simulink model "aocs_plant"  (R2025a)
settings: Solver=ode45  StartTime=0  StopTime=200  RelTol=1e-09  AbsTol=1e-10
undefined symbols (not defined in the file): AOCS, AOCS_Config, AOCS_EnvironmentConfig, AOCS_GNCConfig, AOCS_OrbitConfig, AOCS_SensorConfig, IAU, juliandate, propagateOnboardSgp4
libraries: aerolibtransform2 x8, simulink x8, matrix_library x5
(part 3 of 3)

== system aocs_plant/Flight Dynamics/Orbit & Environment/Environment Products/Atmosphere Products/Atmosphere Model ==
  EnvironmentConfig : Inport  OutDataTypeStr=Bus: EnvironmentConfigBus
  OrbitState : Inport  Port=2  OutDataTypeStr=Bus: OrbitStateBus
  lla : Inport  Port=3  OutDataTypeStr=double
  EnvironmentContext : Inport  Port=4  OutDataTypeStr=Bus: EnvironmentContextBus
  Atmosphere Bus Assembly : BusCreator  Inputs=12  OutDataTypeStr=Bus: AtmosphereBus  NonVirtualBus=on
  Atmosphere Products : Subsystem
  Select Orbit State : BusSelector  OutputSignals=r_I_m,v_I_m_s
  Atmosphere : Outport  OutDataTypeStr=Bus: AtmosphereBus
  wires:
  OrbitState/1 -> Select Orbit State/1
  Atmosphere Bus Assembly/1 -> Atmosphere/1
  Select Orbit State/1 -> Atmosphere Products/1(r_I_m)  "<r_I_m>"
  Select Orbit State/2 -> Atmosphere Products/2(v_I_m_s)  "<v_I_m_s>"
  lla/1 -> Atmosphere Products/3(lla)
  EnvironmentConfig/1 -> Atmosphere Products/4(EnvironmentConfig)
  EnvironmentContext/1 -> Atmosphere Products/5(EnvironmentContext)
  Atmosphere Products/1(rho_kg_m3) -> Atmosphere Bus Assembly/1
  Atmosphere Products/2(rho_raw_kg_m3) -> Atmosphere Bus Assembly/2
  Atmosphere Products/3(rho_uncertainty_1sigma_kg_m3) -> Atmosphere Bus Assembly/3
  Atmosphere Products/4(T_local_K) -> Atmosphere Bus Assembly/4
  Atmosphere Products/5(T_exo_K) -> Atmosphere Bus Assembly/5
  Atmosphere Products/6(n_O_m3) -> Atmosphere Bus Assembly/6
  Atmosphere Products/7(n_N2_m3) -> Atmosphere Bus Assembly/7
  Atmosphere Products/8(n_O2_m3) -> Atmosphere Bus Assembly/8
  Atmosphere Products/9(n_He_m3) -> Atmosphere Bus Assembly/9
  Atmosphere Products/10(n_H_m3) -> Atmosphere Bus Assembly/10
  Atmosphere Products/11(n_N_m3) -> Atmosphere Bus Assembly/11
  Atmosphere Products/12(v_atm_I_m_s) -> Atmosphere Bus Assembly/12

== system aocs_plant/Flight Dynamics/Orbit & Environment/Environment Products/Atmosphere Products/Frame Transformations ==
  In1 : Inport
  In2 : Inport  Port=2
  Clock : Clock
  Clock2 : Clock
  Direction Cosine Matrix ECI to ECEF1 : aerolibtransform2/Direction Cosine Matrix ECI to ECEF  red=IAU-2000/2006  year=2026  month=January  day=1  hour=0  min=0  sec=0  deltaT=Sec  errorflag=Error  extraparamflag=on
      settings: AttributesFormatString=%<red>
  ECI Position to LLA : aerolibtransform2/ECI Position to LLA  red=IAU-2000/2006  year=2026  month=January  day=1  hour=0  min=0  sec=0  deltaT=Sec  errorflag=Error  extraparamflag=on  eunits=Metric (MKS)  earthmodel=WGS84  flat=1/298.257223563  eqradius=6378137
      settings: AttributesFormatString=%<red>
  MATLAB Function : MATLAB Function  TreatAsAtomicUnit=on
  Select Environment Context : BusSelector  OutputSignals=delta_ut1_s,delta_at_s,polar_motion_rad,d_cip_rad
  Select Orbit State : BusSelector  OutputSignals=v_I_m_s,r_I_m
  Terminator : Terminator
  lla : Outport
  v_ECEF_m_s : Outport  Port=2
  C_ECEF_ECI : Outport  Port=3
  wires:
  In2/1 -> Select Environment Context/1
  ECI Position to LLA/1 -> lla/1
  Clock2/1 -> Direction Cosine Matrix ECI to ECEF1/5  "sec"
  Select Environment Context/2 -> Direction Cosine Matrix ECI to ECEF1/2, ECI Position to LLA/3  "<delta_at_s>"
  Select Orbit State/2 -> MATLAB Function/2(r_I_m), ECI Position to LLA/1  "<r_I_m>"
  In1/1 -> Select Orbit State/1
  Select Environment Context/4 -> Direction Cosine Matrix ECI to ECEF1/4, ECI Position to LLA/5  "<d_cip_rad>"
  Select Environment Context/1 -> Direction Cosine Matrix ECI to ECEF1/1, ECI Position to LLA/2  "<delta_ut1_s>"
  Clock/1 -> ECI Position to LLA/6  "sec"
  Select Environment Context/3 -> ECI Position to LLA/4, Direction Cosine Matrix ECI to ECEF1/3  "<polar_motion_rad>"
  Direction Cosine Matrix ECI to ECEF1/1 -> MATLAB Function/3(C_ECEF_ECI), C_ECEF_ECI/1  "C_ECEF_ECI"
  Select Orbit State/1 -> MATLAB Function/1(v_I_m_s)  "<v_I_m_s>"
  MATLAB Function/2(v_ECEF_m_s) -> v_ECEF_m_s/1
  MATLAB Function/1(r_E_m) -> Terminator/1

== system aocs_plant/Flight Dynamics/Orbit & Environment/Orbit Propagator & Time/Orbit State/Orbit Propagator ==
  OrbitAcceleration : Inport
  Bus Creator : BusCreator  Inputs=2
  Orbit Propagator Kepler (unperturbed) : OrbitPropagator  propagator=Numerical (high precision)  accelIn=on  startDate=AOCS_OrbitConfig.epoch_utc  action=None  semiMajorAxis=AOCS_OrbitConfig.semi_major_axis_m  eccentricity=AOCS_OrbitConfig.eccentricity  inclination=AOCS_OrbitConfig.inclination_rad  raan=AOCS_OrbitConfig.raan_rad  argPeriapsis=AOCS_OrbitConfig.argument_of_periapsis_rad  trueAnomaly=AOCS_OrbitConfig.true_anomaly_rad  inertialPosition=[3649700.0 3308200.0 -4676600.0]  inertialVelocity=[-2750.8 6666.4 2573.4]  fixedPosition=[-4142689.0 -2676864.7 -4669861.6]  fixedVelocity=[1452.7 -6720.7 2568.1]  customR=3396200  customMu=4.305e13  customJ2=1.0826269e-03  customOmega=4.06125949e-3  ephemerisStartDate=[2020 1 1 0 0 0]  ephemerisEndDate=[2030 1 1 0 0 0]  useThirdBodyGravity=on  angleUnits=Radians  timeFormat=Gregorian date
  Terminator : Terminator
  OrbitState : Outport  OutDataTypeStr=Bus: OrbitStateBus
  wires:
  Orbit Propagator Kepler (unperturbed)/3 -> Terminator/1
  Bus Creator/1 -> OrbitState/1
  Orbit Propagator Kepler (unperturbed)/1 -> Bus Creator/1  "r_I_m"
  Orbit Propagator Kepler (unperturbed)/2 -> Bus Creator/2  "v_I_m_s"
  OrbitAcceleration/1 -> Orbit Propagator Kepler (unperturbed)/1

== system aocs_plant/Sensors/GNSS/PVT Error Model/Position Error RTN/Gauss-Markov ==
  Innovation Std : Gain  Gain=diag(AOCS_SensorConfig.GNSS.position_gauss_markov_step_std_RTN_m)  Multiplication=Matrix(K*u)
  Innovation W : RandomNumber  Mean=zeros(3,1)  Variance=ones(3,1)  Seed=AOCS_SensorConfig.GNSS.position_gauss_markov_seed  SampleTime=AOCS_SensorConfig.GNSS.sample_time_s
  State Delay : UnitDelay  InitialCondition=zeros(3,1)  SampleTime=AOCS_SensorConfig.GNSS.sample_time_s  HasFrameUpgradeWarning=on
  State Transition : Gain  Gain=AOCS_SensorConfig.GNSS.gauss_markov_alpha
  State Update : Sum
  state : Outport
  wires:
  Innovation W/1 -> Innovation Std/1
  Innovation Std/1 -> State Update/1
  State Delay/1 -> State Transition/1
  State Transition/1 -> State Update/2
  State Update/1 -> State Delay/1, state/1  "state"

== system aocs_plant/Sensors/GNSS/PVT Error Model/Velocity Error RTN/Gauss-Markov ==
  Innovation Std : Gain  Gain=diag(AOCS_SensorConfig.GNSS.velocity_gauss_markov_step_std_RTN_m_s)  Multiplication=Matrix(K*u)
  Innovation W : RandomNumber  Mean=zeros(3,1)  Variance=ones(3,1)  Seed=AOCS_SensorConfig.GNSS.velocity_gauss_markov_seed  SampleTime=AOCS_SensorConfig.GNSS.sample_time_s
  State Delay : UnitDelay  InitialCondition=zeros(3,1)  SampleTime=AOCS_SensorConfig.GNSS.sample_time_s  HasFrameUpgradeWarning=on
  State Transition : Gain  Gain=AOCS_SensorConfig.GNSS.gauss_markov_alpha
  State Update : Sum
  state : Outport
  wires:
  Innovation W/1 -> Innovation Std/1
  Innovation Std/1 -> State Update/1
  State Delay/1 -> State Transition/1
  State Transition/1 -> State Update/2
  State Update/1 -> State Delay/1, state/1  "state"

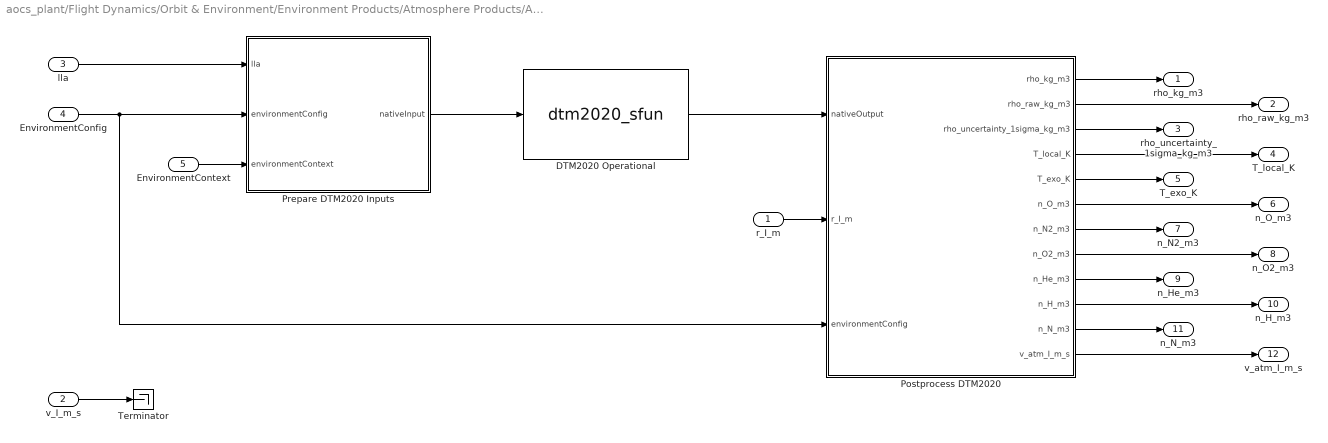
== system aocs_plant/Flight Dynamics/Orbit & Environment/Environment Products/Atmosphere Products/Atmosphere Model/Atmosphere Products ==
  r_I_m : Inport
  v_I_m_s : Inport  Port=2
  lla : Inport  Port=3
  EnvironmentConfig : Inport  Port=4
  EnvironmentContext : Inport  Port=5
  DTM2020 Operational : S-Function  FunctionName=dtm2020_sfun  Parameters=AOCS_DTM2020_CoefficientFile  SFunctionDeploymentMode=off  EnableBusSupport=off
  Postprocess DTM2020 : MATLAB Function  TreatAsAtomicUnit=on
  Prepare DTM2020 Inputs : MATLAB Function  TreatAsAtomicUnit=on
  Terminator : Terminator
  rho_kg_m3 : Outport
  rho_raw_kg_m3 : Outport  Port=2
  rho_uncertainty_1sigma_kg_m3 : Outport  Port=3
  T_local_K : Outport  Port=4
  T_exo_K : Outport  Port=5
  n_O_m3 : Outport  Port=6
  n_N2_m3 : Outport  Port=7
  n_O2_m3 : Outport  Port=8
  n_He_m3 : Outport  Port=9
  n_H_m3 : Outport  Port=10
  n_N_m3 : Outport  Port=11
  v_atm_I_m_s : Outport  Port=12
  wires:
  lla/1 -> Prepare DTM2020 Inputs/1(lla)
  EnvironmentConfig/1 -> Postprocess DTM2020/3(environmentConfig), Prepare DTM2020 Inputs/2(environmentConfig)
  EnvironmentContext/1 -> Prepare DTM2020 Inputs/3(environmentContext)
  Prepare DTM2020 Inputs/1(nativeInput) -> DTM2020 Operational/1
  DTM2020 Operational/1 -> Postprocess DTM2020/1(nativeOutput)
  r_I_m/1 -> Postprocess DTM2020/2(r_I_m)
  Postprocess DTM2020/1(rho_kg_m3) -> rho_kg_m3/1
  Postprocess DTM2020/2(rho_raw_kg_m3) -> rho_raw_kg_m3/1
  Postprocess DTM2020/3(rho_uncertainty_1sigma_kg_m3) -> rho_uncertainty_1sigma_kg_m3/1
  Postprocess DTM2020/4(T_local_K) -> T_local_K/1
  Postprocess DTM2020/5(T_exo_K) -> T_exo_K/1
  Postprocess DTM2020/6(n_O_m3) -> n_O_m3/1
  Postprocess DTM2020/7(n_N2_m3) -> n_N2_m3/1
  Postprocess DTM2020/8(n_O2_m3) -> n_O2_m3/1
  Postprocess DTM2020/9(n_He_m3) -> n_He_m3/1
  Postprocess DTM2020/10(n_H_m3) -> n_H_m3/1
  Postprocess DTM2020/11(n_N_m3) -> n_N_m3/1
  Postprocess DTM2020/12(v_atm_I_m_s) -> v_atm_I_m_s/1
  v_I_m_s/1 -> Terminator/1

== matlab function aocs_plant/Flight Dynamics/Orbit & Environment/Environment Products/Atmosphere Products/Atmosphere Model/Atmosphere Products/Postprocess DTM2020 ==
  data: nativeOutput input; rho_kg_m3 output; r_I_m input; environmentConfig input; rho_raw_kg_m3 output; rho_uncertainty_1sigma_kg_m3 output; T_local_K output; T_exo_K output; n_O_m3 output; n_N2_m3 output; n_O2_m3 output; n_He_m3 output; n_H_m3 output; n_N_m3 output; v_atm_I_m_s output
function [rho_kg_m3, rho_raw_kg_m3, rho_uncertainty_1sigma_kg_m3, ...
    T_local_K, T_exo_K, n_O_m3, n_N2_m3, n_O2_m3, n_He_m3, ...
    n_H_m3, n_N_m3, v_atm_I_m_s] = postprocessDtm(nativeOutput, r_I_m, environmentConfig)
%#codegen
[rho_kg_m3, rho_raw_kg_m3, rho_uncertainty_1sigma_kg_m3, ...
    T_local_K, T_exo_K, n_O_m3, n_N2_m3, n_O2_m3, n_He_m3, ...
    n_H_m3, n_N_m3, v_atm_I_m_s] = dtm2020.postprocessNativeOutput( ...
    nativeOutput, r_I_m, environmentConfig);
end

== matlab function aocs_plant/Sensors/Coarse Sun Sensors/Coarse Sun Sensor Model ==
  data: sun_B_unit input; sun_B_unit_meas output; solar_flux_shadowed_W_m2 input; sun_visibility input; css input; noise_unit input; irradiance_W_m2 output; panel_signals_W_m2 output; valid output
function [sun_B_unit_meas, irradiance_W_m2, panel_signals_W_m2, valid] = coarseSunSensors(sun_B_unit, solar_flux_shadowed_W_m2, sun_visibility, css, noise_unit)
%#codegen
panel_cosines = css.panel_normals_B.' * normalizeVector(sun_B_unit, [1.0; 0.0; 0.0]);
visible = panel_cosines >= css.fov_cos;
ideal_panel_signals_W_m2 = solar_flux_shadowed_W_m2 .* max(panel_cosines, 0.0) .* double(visible);
panel_signals_W_m2 = (1.0 + css.scale_factor) .* ideal_panel_signals_W_m2 + css.bias_W_m2 + css.noise_std_W_m2 .* noise_unit;
panel_signals_W_m2 = min(max(panel_signals_W_m2, 0.0), css.range_W_m2);
if css.resolution_W_m2 > 0.0
    panel_signals_W_m2 = round(panel_signals_W_m2 ./ css.resolution_W_m2) .* css.resolution_W_m2;
end

sun_raw_B = [
    panel_signals_W_m2(1) - panel_signals_W_m2(2);
    panel_signals_W_m2(3) - panel_signals_W_m2(4);
    panel_signals_W_m2(5) - panel_signals_W_m2(6)];
sun_B_unit_meas = normalizeVector(sun_raw_B, [1.0; 0.0; 0.0]);
irradiance_W_m2 = max(panel_signals_W_m2);
valid = double(css.enabled > 0.5 && sun_visibility > 0.5 && irradiance_W_m2 >= css.min_valid_irradiance_W_m2);

if css.mode_id == 2.0
    panel_signals_W_m2 = css.failure_panel_signals_W_m2;
    sun_B_unit_meas = normalizeVector(css.failure_sun_B_unit, [1.0; 0.0; 0.0]);
    irradiance_W_m2 = css.failure_irradiance_W_m2;
    valid = double(css.failure_valid > 0.5);
end

if css.enabled <= 0.5
    panel_signals_W_m2 = zeros(6, 1);
    sun_B_unit_meas = [1.0; 0.0; 0.0];
    irradiance_W_m2 = 0.0;
    valid = 0.0;
end
end

function unitVector = normalizeVector(vector, defaultVector)
normVector = norm(vector);
if normVector <= 1.0e-12
    unitVector = defaultVector;
else
    unitVector = vector ./ normVector;
end
end

== matlab function aocs_plant/Sensors/GNSS/PVT Error Model/Apply RTN Errors ==
  data: rTruth_I_m input; rMeasured_I_m output; vTruth_I_m_s input; positionError_RTN_m input; velocityError_RTN_m_s input; vMeasured_I_m_s output
function [rMeasured_I_m, vMeasured_I_m_s] = applyRtnErrors(rTruth_I_m, vTruth_I_m_s, positionError_RTN_m, velocityError_RTN_m_s)
%#codegen
[rMeasured_I_m, vMeasured_I_m_s] = applyGnssRtnErrors(rTruth_I_m, vTruth_I_m_s, positionError_RTN_m, velocityError_RTN_m_s);
end

== matlab function aocs_plant/Flight Dynamics/Orbit & Environment/Disturbance Torques/Gravity Gradient Path/Gravity Gradient Torque ==
  data: r_I_m input; M_gg_B_Nm output; DCM_be input; I_B input; mu_m3_s2 input
function M_gg_B_Nm = gravityGradientTorque(r_I_m, DCM_be, I_B, mu_m3_s2)
r_norm_m = norm(r_I_m);

if r_norm_m <= 0
    M_gg_B_Nm = zeros(3,1);
    return;
end

r_hat_I = r_I_m / r_norm_m;
r_hat_B = DCM_be * r_hat_I;

M_gg_B_Nm = 3 * mu_m3_s2 / r_norm_m^3 * cross(r_hat_B, I_B * r_hat_B);
end

== matlab function aocs_plant/Flight Dynamics/Orbit & Environment/Disturbance Torques/Aerodynamic Disturbance Path/Relative Wind/Relative Wind Products ==
  data: v_I_m_s input; v_flow_B_m_s output; v_atm_I_m_s input; DCM_be input; rho_kg_m3 input; v_rel_norm_m_s output; q_dyn_N_m2 output
function [v_flow_B_m_s, v_rel_norm_m_s, q_dyn_N_m2] = ...
    relativeWindProducts(v_I_m_s, v_atm_I_m_s, DCM_be, rho_kg_m3)
%#codegen

v_rel_I_m_s = v_I_m_s(:) - v_atm_I_m_s(:);
v_flow_B_m_s = -DCM_be * v_rel_I_m_s;
v_rel_norm_m_s = norm(v_rel_I_m_s);
q_dyn_N_m2 = 0.5 * max(rho_kg_m3, 0.0) * v_rel_norm_m_s^2;
end

== matlab function aocs_plant/Flight Dynamics/Orbit & Environment/Disturbance Torques/Aerodynamic Disturbance Path/Sentman Multispecies Panels ==
  data: v_flow_B_m_s input; F_aero_B_N output; rho_kg_m3 input; T_local_K input; number_densities_m3 input; C_BI input; mass_kg input; aero_enabled input; panel_normals_B input; panel_areas_m2 input; panel_centers_B_m input; wall_temperature_K input; energy_accommodation input; M_aero_B_Nm output; F_aero_I_N output; a_aero_I_m_s2 output; panel_forces_B_N output; q_dyn_N_m2 output
function [F_aero_B_N, M_aero_B_Nm, F_aero_I_N, a_aero_I_m_s2, ...
    panel_forces_B_N, q_dyn_N_m2] = sentmanPanels(v_flow_B_m_s, rho_kg_m3, ...
    T_local_K, number_densities_m3, C_BI, mass_kg, aero_enabled, ...
    panel_normals_B, panel_areas_m2, panel_centers_B_m, ...
    wall_temperature_K, energy_accommodation)
%#codegen
[F_aero_B_N, M_aero_B_Nm, F_aero_I_N, a_aero_I_m_s2, ...
    panel_forces_B_N, q_dyn_N_m2] = computeSentmanPanelAerodynamics( ...
    v_flow_B_m_s, rho_kg_m3, T_local_K, number_densities_m3, C_BI, ...
    mass_kg, aero_enabled, panel_normals_B, panel_areas_m2, ...
    panel_centers_B_m, wall_temperature_K, energy_accommodation);
end

== matlab function aocs_plant/Flight Dynamics/Orbit & Environment/Disturbance Torques/SRP Disturbance Path/SRP Inertial Acceleration ==
  data: F_srp_B_N input; F_srp_I_N output; C_BI input; mass_kg input; a_srp_I_m_s2 output
function [F_srp_I_N, a_srp_I_m_s2] = srpAcceleration(F_srp_B_N, C_BI, mass_kg)
%#codegen
[F_srp_I_N, a_srp_I_m_s2] = computeSrpAcceleration(F_srp_B_N, C_BI, mass_kg);
end

== matlab function aocs_plant/Flight Dynamics/Numerical Checks/Finite Values ==
  data: state input Bus: PlantStateBus; ok output
function ok = finiteState(state)
%#codegen
ok = true;
ok = ok && all(isfinite(state.time_s(:)));
ok = ok && all(isfinite(state.OrbitState.r_I_m(:)));
ok = ok && all(isfinite(state.OrbitState.v_I_m_s(:)));
ok = ok && all(isfinite(state.AttitudeState.euler_rad(:)));
ok = ok && all(isfinite(state.AttitudeState.q_be(:)));
ok = ok && all(isfinite(state.AttitudeState.DCM_be(:)));
ok = ok && all(isfinite(state.AttitudeState.omega_b(:)));
ok = ok && all(isfinite(state.Environment.M_dist_B_Nm(:)));
ok = ok && all(isfinite(state.Environment.B_I_T(:)));
ok = ok && all(isfinite(state.Environment.B_B_T(:)));
ok = ok && all(isfinite(state.Environment.sun_B_unit(:)));
ok = ok && all(isfinite(state.Environment.sun_I_unit(:)));
ok = ok && all(isfinite(state.Environment.r_sun_I_m(:)));
ok = ok && all(isfinite(state.Environment.sun_distance_m(:)));
ok = ok && all(isfinite(state.Environment.solar_flux_W_m2(:)));
ok = ok && all(isfinite(state.Environment.solar_flux_shadowed_W_m2(:)));
ok = ok && all(isfinite(state.Environment.sun_visibility(:)));
ok = ok && all(isfinite(state.Environment.Atmosphere.rho_kg_m3(:)));
ok = ok && all(isfinite(state.Environment.Atmosphere.rho_raw_kg_m3(:)));
ok = ok && all(isfinite(state.Environment.Atmosphere.rho_uncertainty_1sigma_kg_m3(:)));
ok = ok && all(isfinite(state.Environment.Atmosphere.T_local_K(:)));
ok = ok && all(isfinite(state.Environment.Atmosphere.T_exo_K(:)));
ok = ok && all(isfinite(state.Environment.Atmosphere.n_O_m3(:)));
ok = ok && all(isfinite(state.Environment.Atmosphere.n_N2_m3(:)));
ok = ok && all(isfinite(state.Environment.Atmosphere.n_O2_m3(:)));
ok = ok && all(isfinite(state.Environment.Atmosphere.n_He_m3(:)));
ok = ok && all(isfinite(state.Environment.Atmosphere.n_H_m3(:)));
ok = ok && all(isfinite(state.Environment.Atmosphere.n_N_m3(:)));
ok = ok && all(isfinite(state.Environment.Atmosphere.v_atm_I_m_s(:)));
ok = ok && all(isfinite(state.Environment.M_srp_B_Nm(:)));
ok = ok && all(isfinite(state.Environment.F_srp_B_N(:)));
ok = ok && all(isfinite(state.Environment.F_srp_I_N(:)));
ok = ok && all(isfinite(state.Environment.a_srp_I_m_s2(:)));
ok = ok && all(isfinite(state.Environment.M_aero_B_Nm(:)));
ok = ok && all(isfinite(state.Environment.F_aero_B_N(:)));
ok = ok && all(isfinite(state.Environment.F_aero_I_N(:)));
ok = ok && all(isfinite(state.Environment.a_aero_I_m_s2(:)));
ok = ok && all(isfinite(state.Environment.a_dist_I_m_s2(:)));
ok = ok && all(isfinite(state.Environment.q_dyn_N_m2(:)));
ok = ok && all(isfinite(state.Environment.v_rel_norm_m_s(:)));
end

== matlab function aocs_plant/Flight Dynamics/Orbit & Environment/Orbit Propagator & Time/Orbit and Time Context/MATLAB Function ==
  data: epoch_utc input; dyear output; t_s input
function dyear = decimalYearUtc(epoch_utc, t_s)
year = floor(epoch_utc(1));
month = floor(epoch_utc(2));
day = floor(epoch_utc(3));
hour = floor(epoch_utc(4));
minute = floor(epoch_utc(5));
second = epoch_utc(6);

monthStart = [0 31 59 90 120 151 181 212 243 273 304 334];
leap = (mod(year,4)==0 && mod(year,100)~=0) || mod(year,400)==0;

leapOffset = 0;
if leap && month > 2
    leapOffset = 1;
end

secIntoYear = (monthStart(month) + leapOffset + day - 1) * 86400 ...
    + hour * 3600 + minute * 60 + second + t_s;

dyear = year + secIntoYear / ((365 + double(leap)) * 86400);
end

== matlab function aocs_plant/Flight Dynamics/Orbit & Environment/Environment Products/Atmosphere Products/Frame Transformations/MATLAB Function ==
  data: v_I_m_s input; r_I_m input; C_ECEF_ECI input; r_E_m output; v_ECEF_m_s output
function [r_E_m, v_ECEF_m_s] = eciStateToEcefState(v_I_m_s, r_I_m, C_ECEF_ECI)
%#codegen

omega_E_rad_s = 7.2921150e-5;
omega_E_ECEF_rad_s = [0; 0; omega_E_rad_s];

r_E_m = C_ECEF_ECI * r_I_m;
v_E_raw_m_s = C_ECEF_ECI * v_I_m_s;

v_ECEF_m_s = v_E_raw_m_s - cross(omega_E_ECEF_rad_s, r_E_m);
end

== matlab function aocs_plant/Sensors/Gyro/Gyro Calibration ==
  data: omega_b_rad_s input; omega_cal_rad_s output; gyro input
function omega_cal_rad_s = applyGyroCalibration(omega_b_rad_s, gyro)
%#codegen
S = eye(3) + diag(gyro.scale_factor);
omega_cal_rad_s = gyro.misalignment_matrix * S * omega_b_rad_s;
end

== matlab function aocs_plant/Flight Dynamics/Orbit & Environment/Environment Products/Sun Products/Sun Geometry ==
  data: r_sun_I_m_ephem input size=[3 1]; sun_B_unit output size=[3 1]; solar_constant_W_m2 input size=1; r_I_m input size=[3 1]; DCM_be input size=[3 3]; sun_I_unit output size=[3 1]; r_sun_I_m output size=[3 1]; sun_distance_m output size=1; solar_flux_W_m2 output size=1
function [sun_B_unit, sun_I_unit, r_sun_I_m, sun_distance_m, solar_flux_W_m2] = sunProducts(r_sun_I_m_ephem, solar_constant_W_m2, r_I_m, DCM_be)
%#codegen
sun_B_unit = zeros(3, 1);
sun_I_unit = zeros(3, 1);
r_sun_I_m = zeros(3, 1);
sun_distance_m = 0.0;
solar_flux_W_m2 = 0.0;
[sun_B_unit, sun_I_unit, r_sun_I_m, sun_distance_m, solar_flux_W_m2] = ...
 computeSunProducts(r_sun_I_m_ephem, solar_constant_W_m2, r_I_m, DCM_be);
end

== matlab function aocs_plant/Flight Dynamics/Orbit & Environment/Environment Products/Solar Radiation Pressure/MATLAB Function ==
  data: sun_B_unit input size=[3 1]; M_srp_B_Nm output size=[3 1]; solar_flux_shadowed_W_m2 input size=1; srp_enabled input size=1; srp_area_ref_m2 input size=1; srp_coefficient_reflectivity input size=1; srp_center_of_pressure_B_m input size=[3 1]; F_srp_B_N output size=[3 1]; P_srp_N_m2 output size=1
function [M_srp_B_Nm, F_srp_B_N, P_srp_N_m2] = fcn(sun_B_unit, solar_flux_shadowed_W_m2, srp_enabled, srp_area_ref_m2, srp_coefficient_reflectivity, srp_center_of_pressure_B_m)
%#codegen

[M_srp_B_Nm, F_srp_B_N, P_srp_N_m2] = computeSrpTorque( ...
 sun_B_unit, solar_flux_shadowed_W_m2, srp_enabled, ...
 srp_area_ref_m2, srp_coefficient_reflectivity, srp_center_of_pressure_B_m);
end

== matlab function aocs_plant/Flight Dynamics/Orbit & Environment/Environment Products/Geomagnetic Field Model/LLA to IGRF Inputs ==
  data: lla input; h_m output; lat_deg output; lon_deg output
function [h_m, lat_deg, lon_deg] = llaToIgrfInputs(lla)
lat_deg = lla(1);
lon_deg = lla(2);
h_m = lla(3);
end

== matlab function aocs_plant/Flight Dynamics/Orbit & Environment/Environment Products/Atmosphere Products/Atmosphere Model/Atmosphere Products/Prepare DTM2020 Inputs ==
  data: lla input; nativeInput output; environmentConfig input; environmentContext input
function nativeInput = prepareDtmInputs(lla, environmentConfig, environmentContext)
%#codegen
nativeInput = dtm2020.prepareNativeInput(lla, environmentConfig, environmentContext);
end

== matlab function aocs_plant/Sensors/Magnetometer/Magnetometer Calibration ==
  data: B_B_T input; B_cal_T output; magnetometer input
function B_cal_T = applyMagnetometerCalibration(B_B_T, magnetometer)
%#codegen
S = eye(3) + diag(magnetometer.scale_factor);
B_cal_T = magnetometer.misalignment_matrix * S * B_B_T;
end
